simulink model "PIDRover"  (R2021a)
settings: Solver=VariableStepAuto  StartTime=0.0  StopTime=100  RelTol=1e-5
libraries: slpidlib x2
settings Model: Creator=templ  LastModifiedBy=templ
settings DataIOCC: ReturnWorkspaceOutputs=off

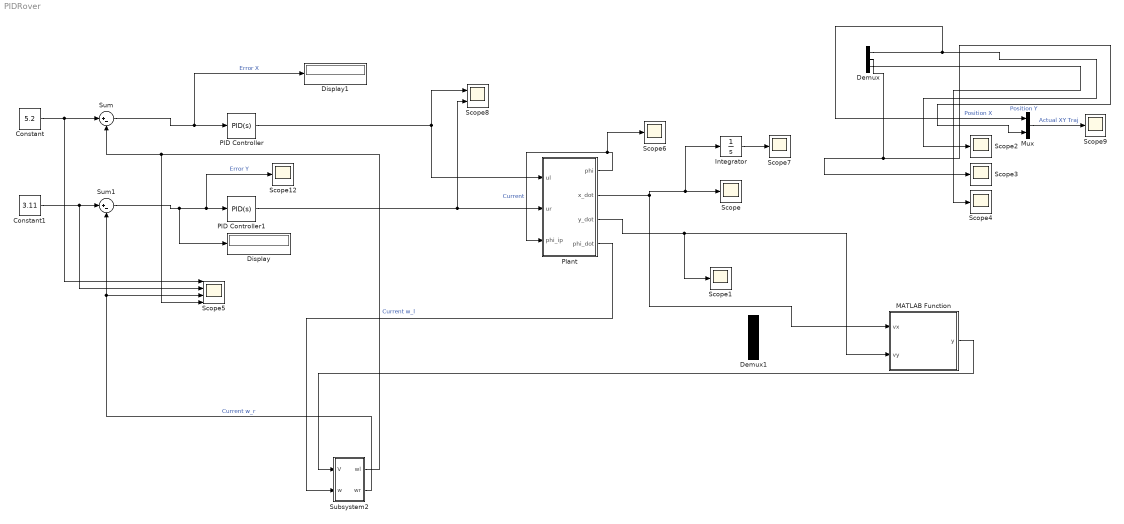
== system PIDRover ==
  Constant : Constant  Value=5.2
  Constant1 : Constant  Value=3.11
  Demux : Demux  Outputs=3
  Demux1 : Demux  Outputs=3
  Display : Display
  Display1 : Display
  Integrator : Integrator
  MATLAB Function : MATLAB Function  TreatAsAtomicUnit=on
  Mux : Mux  Inputs=2
  PID Controller : slpidlib/PID Controller  Controller=PID  Form=Parallel  TimeDomain=Continuous-time  UseExternalTs=off  SampleTime=-1  IntegratorMethod=Forward Euler  FilterMethod=Forward Euler  ControllerParametersSource=internal  P=10  I=1  D=5  UseFilter=on  N=100  TunerSelectOption=Transfer Function Based (PID Tuner App)  InitialConditionSource=internal  InitialConditionForIntegrator=0  InitialConditionForFilter=0  DifferentiatorICPrevScaledInput=0  ExternalReset=none  TrackingMode=off  Kt=1  LimitOutput=off  SatLimitsSource=internal  UpperSaturationLimit=inf  LowerSaturationLimit=-inf  LinearizeAsGain=on  AntiWindupMode=none  Kb=1  POutMin=[]  POutMax=[]  IOutMin=[]  IOutMax=[]  DOutMin=[]  DOutMax=[]  NOutMin=[]  NOutMax=[]  SumOutMin=[]  SumOutMax=[]  SaturationOutMin=[]  SaturationOutMax=[]  PParamMin=[]  PParamMax=[]  IParamMin=[]  IParamMax=[]  DParamMin=[]  DParamMax=[]  NParamMin=[]  NParamMax=[]  KbParamMin=[]  KbParamMax=[]  KtParamMin=[]  KtParamMax=[]  KbOutMin=[]  KbOutMax=[]  KtOutMin=[]  KtOutMax=[]  IntegratorOutMin=[]  IntegratorOutMax=[]  FilterOutMin=[]  FilterOutMax=[]  SumI1OutMin=[]  SumI1OutMax=[]  SumI2OutMin=[]  SumI2OutMax=[]  SumI3OutMin=[]  SumI3OutMax=[]  SumI4OutMin=[]  SumI4OutMax=[]  SumDOutMin=[]  SumDOutMax=[]  DifferentiatorOutMin=[]  DifferentiatorOutMax=[]  FilterDiffOutCoefMin=[]  FilterDiffOutCoefMax=[]  ReciprocalOutMin=[]  ReciprocalOutMax=[]  SumDenOutMin=[]  SumDenOutMax=[]  SumNumOutMin=[]  SumNumOutMax=[]  DivideOutMin=[]  DivideOutMax=[]  UdiffTsProdOutMin=[]  UdiffTsProdOutMax=[]  NTsProdOutMin=[]  NTsProdOutMax=[]  UintegralTsProdOutMin=[]  UintegralTsProdOutMax=[]  UngainTsProdOutMin=[]  UngainTsProdOutMax=[]  IntegratorContinuousStateAttributes=''  IntegratorStateMustResolveToSignalObject=off  IntegratorRTWStateStorageClass=Auto  FilterContinuousStateAttributes=''  FilterStateMustResolveToSignalObject=off  FilterRTWStateStorageClass=Auto  ParallelPVariant=InternalParameters  IdealPVariant=Disabled  IVariant=InternalParameters  DVariant=InternalParameters  IntegratorVariant=Continuous  SatVariant=Disabled  AWVariant=Passthrough  PCopyVariant=Disabled  TRVariant=Disabled  FdbkBlocksVariant=Forward  IdealPFdbkVariant=Disabled  SatFdbkVariant=Disabled  DerivativeFilterVariant=ContFilter  NVariant=InternalParameters  NCopyVariant=Disabled  FilterICVariant=InternalICsFilter  IntegratorICVariant=InternalICs  ExternalResetVariant=Disabled  TRSumVariant=Passthrough  SumFdbkVariant=Disabled  SumVariant=Sum_PID  TsampFilterVariant=InternalTs  TsampNgainVariant=Passthrough  TsampIntegralVariant=Passthrough  ExternalSaturationOutDataTypeStr=Inherit: Same as second input
  PID Controller1 : slpidlib/PID Controller  Controller=PID  Form=Parallel  TimeDomain=Continuous-time  UseExternalTs=off  SampleTime=-1  IntegratorMethod=Forward Euler  FilterMethod=Forward Euler  ControllerParametersSource=internal  P=10  I=1  D=5  UseFilter=on  N=100  TunerSelectOption=Transfer Function Based (PID Tuner App)  InitialConditionSource=internal  InitialConditionForIntegrator=0  InitialConditionForFilter=0  DifferentiatorICPrevScaledInput=0  ExternalReset=none  TrackingMode=off  Kt=1  LimitOutput=off  SatLimitsSource=internal  UpperSaturationLimit=inf  LowerSaturationLimit=-inf  LinearizeAsGain=on  AntiWindupMode=none  Kb=1  POutMin=[]  POutMax=[]  IOutMin=[]  IOutMax=[]  DOutMin=[]  DOutMax=[]  NOutMin=[]  NOutMax=[]  SumOutMin=[]  SumOutMax=[]  SaturationOutMin=[]  SaturationOutMax=[]  PParamMin=[]  PParamMax=[]  IParamMin=[]  IParamMax=[]  DParamMin=[]  DParamMax=[]  NParamMin=[]  NParamMax=[]  KbParamMin=[]  KbParamMax=[]  KtParamMin=[]  KtParamMax=[]  KbOutMin=[]  KbOutMax=[]  KtOutMin=[]  KtOutMax=[]  IntegratorOutMin=[]  IntegratorOutMax=[]  FilterOutMin=[]  FilterOutMax=[]  SumI1OutMin=[]  SumI1OutMax=[]  SumI2OutMin=[]  SumI2OutMax=[]  SumI3OutMin=[]  SumI3OutMax=[]  SumI4OutMin=[]  SumI4OutMax=[]  SumDOutMin=[]  SumDOutMax=[]  DifferentiatorOutMin=[]  DifferentiatorOutMax=[]  FilterDiffOutCoefMin=[]  FilterDiffOutCoefMax=[]  ReciprocalOutMin=[]  ReciprocalOutMax=[]  SumDenOutMin=[]  SumDenOutMax=[]  SumNumOutMin=[]  SumNumOutMax=[]  DivideOutMin=[]  DivideOutMax=[]  UdiffTsProdOutMin=[]  UdiffTsProdOutMax=[]  NTsProdOutMin=[]  NTsProdOutMax=[]  UintegralTsProdOutMin=[]  UintegralTsProdOutMax=[]  UngainTsProdOutMin=[]  UngainTsProdOutMax=[]  IntegratorContinuousStateAttributes=''  IntegratorStateMustResolveToSignalObject=off  IntegratorRTWStateStorageClass=Auto  FilterContinuousStateAttributes=''  FilterStateMustResolveToSignalObject=off  FilterRTWStateStorageClass=Auto  ParallelPVariant=InternalParameters  IdealPVariant=Disabled  IVariant=InternalParameters  DVariant=InternalParameters  IntegratorVariant=Continuous  SatVariant=Disabled  AWVariant=Passthrough  PCopyVariant=Disabled  TRVariant=Disabled  FdbkBlocksVariant=Forward  IdealPFdbkVariant=Disabled  SatFdbkVariant=Disabled  DerivativeFilterVariant=ContFilter  NVariant=InternalParameters  NCopyVariant=Disabled  FilterICVariant=InternalICsFilter  IntegratorICVariant=InternalICs  ExternalResetVariant=Disabled  TRSumVariant=Passthrough  SumFdbkVariant=Disabled  SumVariant=Sum_PID  TsampFilterVariant=InternalTs  TsampNgainVariant=Passthrough  TsampIntegralVariant=Passthrough  ExternalSaturationOutDataTypeStr=Inherit: Same as second input
  Plant : Subsystem
  Scope{,1..4,6..7,9,12} (9 alike) : Scope
  Scope5 : Scope  NumInputPorts=4
  Scope8 : Scope  NumInputPorts=2
  Subsystem2 : Subsystem
  Sum : Sum  Inputs=|+-
  Sum1 : Sum  Inputs=|+-
  wires:
  Demux/1 -> Mux/1, Scope2/1  "Position X"
  Demux/2 -> Scope3/1, Mux/2  "Position Y"
  Demux/3 -> Scope4/1
  Mux/1 -> Scope9/1  "Actual XY Traj"
  Constant/1 -> Scope5/1, Sum/1
  Sum/1 -> Display1/1, PID Controller/1  "Error X"
  Constant1/1 -> Scope5/2, Sum1/1
  Sum1/1 -> Display/1, Scope12/1, PID Controller1/1  "Error Y"
  PID Controller/1 -> Plant/1(ul), Scope8/1
  PID Controller1/1 -> Scope8/2, Plant/2(ur)
  MATLAB Function/1(y) -> Subsystem2/1(V)
  Subsystem2/1(wl) -> Scope5/4, Sum/2  "Current w_l"
  Subsystem2/2(wr) -> Sum1/2, Scope5/3  "Current w_r"
  Plant/2(x_dot) -> MATLAB Function/1(vx), Integrator/1, Scope/1
  Plant/3(y_dot) -> Scope1/1, MATLAB Function/2(vy)
  Plant/1(phi) -> Scope6/1, Plant/3(phi_ip)  "Current"
  Plant/4(phi_dot) -> Subsystem2/2(w)
  Integrator/1 -> Scope7/1

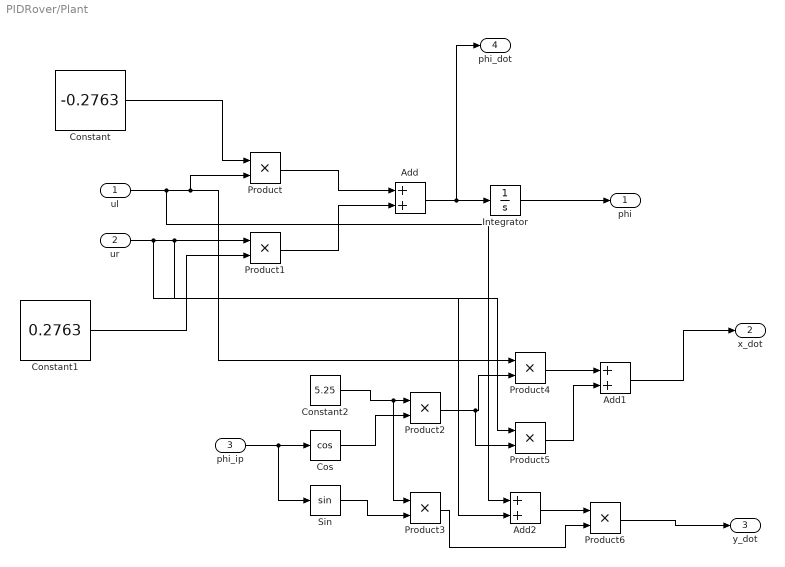
== system PIDRover/Plant ==
  ul : Inport
  ur : Inport  Port=2
  phi_ip : Inport  Port=3
  Add : Sum
  Add1 : Sum
  Add2 : Sum
  Constant : Constant  Value=-0.2763
  Constant1 : Constant  Value=0.2763
  Constant2 : Constant  Value=5.25
  Cos : Trigonometry  Operator=cos
  Integrator : Integrator
  Product{,1..6} (7 alike) : Product
  Sin : Trigonometry
  phi : Outport
  x_dot : Outport  Port=2
  y_dot : Outport  Port=3
  phi_dot : Outport  Port=4
  wires:
  ur/1 -> Add2/2, Product5/1, Product1/1
  Product/1 -> Add/1
  Integrator/1 -> phi/1
  Product1/1 -> Add/2
  Constant1/1 -> Product1/2
  Add/1 -> phi_dot/1, Integrator/1
  ul/1 -> Add2/1, Product4/1, Product/2
  Constant/1 -> Product/1
  phi_ip/1 -> Sin/1, Cos/1
  Cos/1 -> Product2/2
  Constant2/1 -> Product3/1, Product2/1
  Sin/1 -> Product3/2
  Product2/1 -> Product5/2, Product4/2
  Product4/1 -> Add1/1
  Product5/1 -> Add1/2
  Add1/1 -> x_dot/1
  Add2/1 -> Product6/1
  Product3/1 -> Product6/2
  Product6/1 -> y_dot/1

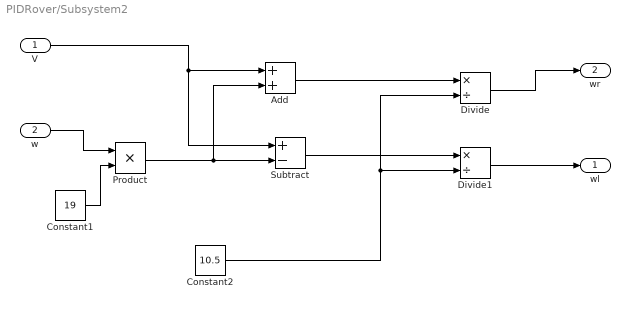
== system PIDRover/Subsystem2 ==
  V : Inport
  w : Inport  Port=2
  Add : Sum
  Constant1 : Constant  Value=19
  Constant2 : Constant  Value=10.5
  Divide : Product  Inputs=*/
  Divide1 : Product  Inputs=*/
  Product : Product
  Subtract : Sum  Inputs=+-
  wl : Outport
  wr : Outport  Port=2
  wires:
  V/1 -> Subtract/1, Add/1
  Add/1 -> Divide/1
  Constant2/1 -> Divide1/2, Divide/2
  Subtract/1 -> Divide1/1
  Product/1 -> Subtract/2, Add/2
  Divide1/1 -> wl/1
  Divide/1 -> wr/1
  Constant1/1 -> Product/2
  w/1 -> Product/1

== matlab function PIDRover/MATLAB Function ==
  data: vx input; y output; vy input
function y = fcn(vx,vy)
vnet=sqrt((vx^2)+(vy^2));



y = vnet;
